simulink model "modelo_bateria_examen"  (R2021b)
settings: Solver=daessc  StartTime=0.0  StopTime=30000  RelTol=1e-3
InitFcn:
  | MaxCellVoltage=340;
undefined symbols (not defined in the file): Ion, Lithium
libraries: spsBreakerLib x2, spsBatteryLib x1, spsControlledCurrentSourceLib x1, spsControlledVoltageSourceLib x1, spspowerguiLib x1
settings Model: Creator=Usuario_UMA  LastModifiedBy=Daniel
settings SolverCC: ZeroCrossAlgorithm=Adaptive  AlgebraicLoopSolver=LineSearch
settings DebuggingCC: IgnoredZcDiagnostic=none  SFMachineParentedDataDiag=warning

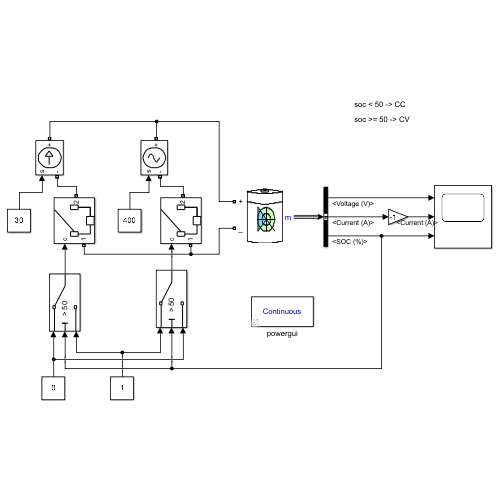
[thumbnail: Simulink's stored preview of the top-level diagram]
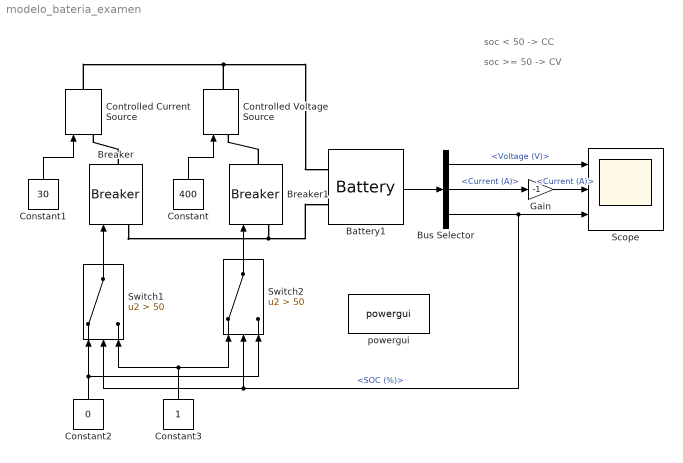
== system modelo_bateria_examen ==
  note: soc < 50 -> CC
  note: soc >= 50 -> CV
  Battery1 : spsBatteryLib/Battery  BatType=Lithium-Ion  ShowTempParam=off  ThermalPreset=no  ShowAgeParam=off  NomV=340  NomQ=170  SOC=10  Batt_Tr=30  PresetModel=on  MaxQ=170  MinV=255  FullV=395.7556  Dis_rate=73.913  R=0.02  Normal_OP=153.7391  expZone="[367.3312      8.352174]"  current=[6.5 13 32.5]  Units=Time  Tci=20  NomT=20  T2=-30  MaxQ2=4.8  FullV2=7.1  Normal_OP2=5.655  expZone2="[6.58           1]"  Rca=0.6  ti=2000  Dp=0  Neq0=0  Tsim=1e6  Ta1=25  Qeol=5.4*0.9  Reol=0.013333*1.2  Char_age=[2.3478, 3]  Dis_age=[2.3478, 10]  N1=1500  N2=10500  N3=1000  N4=1400  Ta2=45  N5=950
  Breaker : spsBreakerLib/Breaker  InitialState=0  SwitchingTimes="[1/60  5/60]"  External=on  BreakerResistance=0.01  SnubberResistance=1e6  SnubberCapacitance=inf  Measurements=None  MoreParameters=on  NoBreakLoop=off
      settings: SourceProductBaseCode=PS
  Breaker1 : spsBreakerLib/Breaker  InitialState=0  SwitchingTimes="[1/60  5/60]"  External=on  BreakerResistance=0.01  SnubberResistance=1e6  SnubberCapacitance=inf  Measurements=None  MoreParameters=on  NoBreakLoop=off
      settings: SourceProductBaseCode=PS
  Bus Selector : BusSelector  OutputSignals=Voltage (V),Current (A),SOC (%)
  Constant : Constant  Value=400
  Constant1 : Constant  Value=30  SampleTime=-1
  Constant2 : Constant  Value=0  SampleTime=-1
  Constant3 : Constant  SampleTime=-1
  Controlled Current Source : spsControlledCurrentSourceLib/Controlled Current Source  Initialize=on  Source_Type=AC  Amplitude=0  Phase=0  Frequency=0  Measurements=None
  Controlled Voltage Source : spsControlledVoltageSourceLib/Controlled Voltage Source  Initialize=on  Source_Type=AC  Amplitude=0  Phase=0  Frequency=0  Measurements=None
  Gain : Gain  Gain=-1
  Scope : Scope  NumInputPorts=3
  Switch1 : Switch  Criteria=u2 > Threshold  Threshold=50
  Switch2 : Switch  Criteria=u2 > Threshold  Threshold=50
  powergui : spspowerguiLib/powergui  Priority=1  SimulationMode=Continuous  SampleTime=50e-6  frequency=60  Iterations=50  frequencyindice=0  Pbase=100e6  ErrMax=1e-4  UnitsV=kV  UnitsW=MW  buscounter=0  FunctionMessages=off  echomessages=off  EnableUseOfTLC=off  CurrentSourceSwitches=off  DisableSnubberDevices=off  DisableRonSwitches=off  DisableVfSwitches=off  DisplayEquations=off  AutomaticDiscreteSolvers=off  SolverType=Tustin/Backward Euler (TBE)  Interpol=off  ExternalGateDelay=off  methode=off  Ts=100  x0status=blocks  SPID=on  SwTol=0  HookPort=off  NonlinearTolerance=1e-4  nMaxIteration=100  ContinueOnMaxIteration=off  RestoreLinks=warning  ResistiveCurrentMeasurement=off  Frange=[0:2:500]  Ylog=off  Xlog=on  ShowGrid=off  save=off  variable=ZData  structure=0  ZoomFFT=off  StartTime=0.0  cycles=1  DisplayStyle=1  fundamental=60  FreqAxis=off  MaxFrequency=1000  frequencyindicesteady=1  RmsSteady=1  display=off
  wires:
  Battery1/1 -> Bus Selector/1
  Bus Selector/1 -> Scope/1  "<Voltage (V)>"
  Bus Selector/3 -> Scope/3, Switch2/2, Switch1/2  "<SOC (%)>"
  Constant/1 -> Controlled Voltage Source/1
  Constant2/1 -> Switch1/1, Switch2/3
  Constant3/1 -> Switch2/1, Switch1/3
  Switch2/1 -> Breaker1/1
  Constant1/1 -> Controlled Current Source/1
  Switch1/1 -> Breaker/1
  Gain/1 -> Scope/2  "<Current (A)>"
  Bus Selector/2 -> Gain/1  "<Current (A)>"
  connections:
  Breaker1/LConn1 -- Battery1/LConn2 -- Breaker/LConn1
  Controlled Voltage Source/RConn1 -- Battery1/LConn1 -- Controlled Current Source/RConn1
  Breaker1/RConn1 -- Controlled Voltage Source/LConn1
  Breaker/RConn1 -- Controlled Current Source/LConn1
